simulink model "lab2_EmulationPID"  (R2020b)
settings: Solver=VariableStepAuto  StartTime=0.0  StopTime=10.0  RelTol=1e-3
undefined symbols (not defined in the file): denCdExact, denCdFE, denCdTustin, DiscIntNeverNeededParam, drv, enable_BlackBox, gbox, Kd, Ki, Kp, mld, mot, numCdExact, numCdFE, numCdTustin, rads2rpm, sens, stepAmplitude, tau_sf_hat_final, Tl, Ts
settings Model: Creator=Musta  LastModifiedBy=Musta

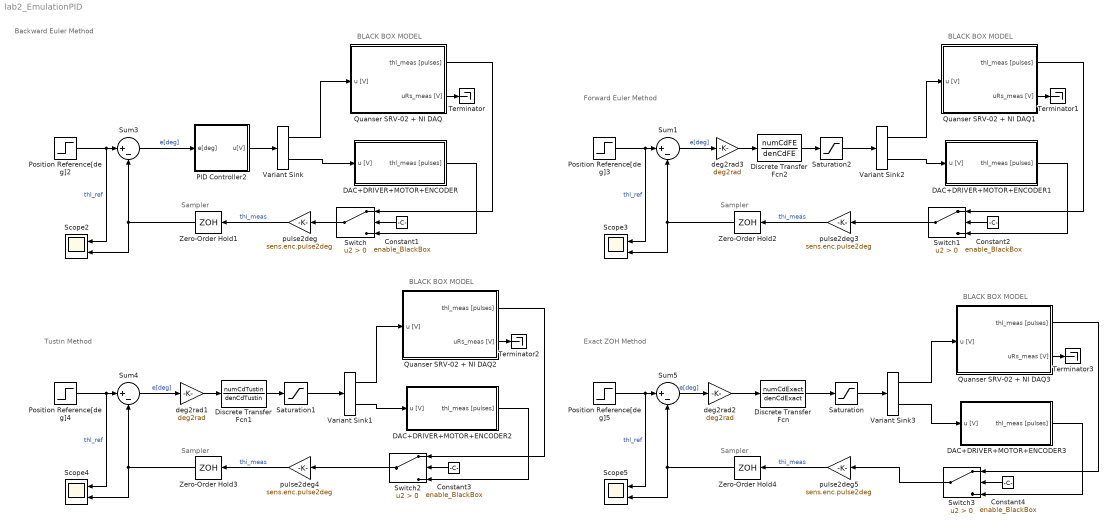
== system lab2_EmulationPID ==
  note: Tustin Method
  note: Sampler
  note: Sampler
  note: Forward Euler Method
  note: Backward Euler Method
  note: Sampler
  note: Sampler
  note: Exact ZOH Method
  note: BLACK BOX MODEL
  note: BLACK BOX MODEL
  note: BLACK BOX MODEL
  note: BLACK BOX MODEL
  Constant{1..4} (4 alike) : Constant  Value=enable_BlackBox
  DAC+DRIVER+MOTOR+ENCODER : Subsystem
  DAC+DRIVER+MOTOR+ENCODER1 : Subsystem
  DAC+DRIVER+MOTOR+ENCODER2 : Subsystem
  DAC+DRIVER+MOTOR+ENCODER3 : Subsystem
  Discrete Transfer Fcn : DiscreteTransferFcn  Numerator=numCdExact  Denominator=denCdExact  SampleTime=Ts
  Discrete Transfer Fcn1 : DiscreteTransferFcn  Numerator=numCdTustin  Denominator=denCdTustin  SampleTime=Ts
  Discrete Transfer Fcn2 : DiscreteTransferFcn  Numerator=numCdFE  Denominator=denCdFE  SampleTime=Ts
  PID Controller2 : Subsystem
  Position Reference[deg]{2..5} (4 alike) : Step  Time=0  After=stepAmplitude  SampleTime=0
  Quanser SRV-02 + NI DAQ : Subsystem  mask(Quanser SRV-02 (with inertial load) + NI DAQ){Ts=Ts, fricType=Karnopp}
      mask prompts: Ts "NI DAQ Sample Time:"; fricType "Friction model"
      mask help: Quanser SRV-02 (with inertial load) + NI DAQ model.
      mask init:
      | %%  Sensors data
      | 
      | %   shunt resistor
      | sens.curr.Rs = 0.5;                         %   resistance [Ohm]   
      | sens.curr.uRs_std = 0.01;                   %   voltage noise standard dev [V]                           
      | sens.curr.uRs_var = sens.curr.uRs_std^2;	%   voltage noise variance [V^2]
      | 
      | %   Hewlett-Packard HEDS-5540#A06 optical encoder
      | sens.enc.ppr = 500*4;                       %   pulses per rotation
      | sens.enc.pulse2deg = 360/sens.enc.ppr;      %   [pulses] -> [deg]
      | sens.enc.pulse2rad = 2*pi/sens.enc.ppr;     %   [pulses] -> [rad]
      | sens.enc.deg2pulse = sens.enc.ppr/360;      %   [deg] -> [pulses]
      | sens.enc.rad2pulse = sens.enc.ppr/2/pi;     %   [rad] -> [pulses]
      | 
      | 
      | %%  Data acquisition board (daq) data
      | 
      | %   NI PCI-6221 DAC data
      | daq.dac.bits = 16;                                  %   resolution (bits)
      | daq.dac.fs   = 10;                                  %   full scale 
      | daq.dac.q    = 2*daq.dac.fs/(2^daq.dac.bits-1);     %	quantization
      | 
      | %   NI PCI-6221 ADC data
      | daq.adc.bits = 16;                                  %   resolution (bits)
      | daq.adc.fs   = 10;                                  %   full scale (as set in SLDRT Analog Input block)
      | daq.adc.q    = 2*daq.adc.fs/(2^daq.adc.bits-1);     %   quantization
      mask Help:
      | Riccardo Antonello (antonello@dei.unipd.it)
      | 
      | April 24, 2020
      | 
      | Dept. of Information Engineering, University of Padova
      mask TypeOptions fricType: Coulomb + viscous | Karnopp
  Quanser SRV-02 + NI DAQ1 : Subsystem  mask(Quanser SRV-02 (with inertial load) + NI DAQ){Ts=Ts, fricType=Karnopp}
      mask prompts: Ts "NI DAQ Sample Time:"; fricType "Friction model"
      mask help: Quanser SRV-02 (with inertial load) + NI DAQ model.
      mask init: same as lab2_EmulationPID/Quanser SRV-02 + NI DAQ
      mask Help:
      | Riccardo Antonello (antonello@dei.unipd.it)
      | 
      | April 24, 2020
      | 
      | Dept. of Information Engineering, University of Padova
      mask TypeOptions fricType: Coulomb + viscous | Karnopp
  Quanser SRV-02 + NI DAQ2 : Subsystem  mask(Quanser SRV-02 (with inertial load) + NI DAQ){Ts=Ts, fricType=Karnopp}
      mask prompts: Ts "NI DAQ Sample Time:"; fricType "Friction model"
      mask help: Quanser SRV-02 (with inertial load) + NI DAQ model.
      mask init: same as lab2_EmulationPID/Quanser SRV-02 + NI DAQ
      mask Help:
      | Riccardo Antonello (antonello@dei.unipd.it)
      | 
      | April 24, 2020
      | 
      | Dept. of Information Engineering, University of Padova
      mask TypeOptions fricType: Coulomb + viscous | Karnopp
  Quanser SRV-02 + NI DAQ3 : Subsystem  mask(Quanser SRV-02 (with inertial load) + NI DAQ){Ts=Ts, fricType=Karnopp}
      mask prompts: Ts "NI DAQ Sample Time:"; fricType "Friction model"
      mask help: Quanser SRV-02 (with inertial load) + NI DAQ model.
      mask init: same as lab2_EmulationPID/Quanser SRV-02 + NI DAQ
      mask Help:
      | Riccardo Antonello (antonello@dei.unipd.it)
      | 
      | April 24, 2020
      | 
      | Dept. of Information Engineering, University of Padova
      mask TypeOptions fricType: Coulomb + viscous | Karnopp
  Saturation : Saturate  UpperLimit=10  LowerLimit=-10
  Saturation1 : Saturate  UpperLimit=10  LowerLimit=-10
  Saturation2 : Saturate  UpperLimit=10  LowerLimit=-10
  Scope{2..5} (4 alike) : Scope  NumInputPorts=2
  Sum{1,3..5} (4 alike) : Sum  Inputs=|+-
  Switch{,1..3} (4 alike) : Switch  Criteria=u2 > Threshold
  Terminator{,1..3} (4 alike) : Terminator
  Variant Sink{,1..3} (4 alike) : VariantSink
  Zero-Order Hold{1..4} (4 alike) : ZeroOrderHold  SampleTime=Ts
  deg2rad1 : Gain  Gain=deg2rad
  deg2rad2 : Gain  Gain=deg2rad
  deg2rad3 : Gain  Gain=deg2rad
  pulse2deg{,3..5} (4 alike) : Gain  Gain=sens.enc.pulse2deg
  wires:
  Position Reference[deg]3/1 -> Scope3/1, Sum1/1  "thl_ref"
  Position Reference[deg]5/1 -> Scope5/1, Sum5/1  "thl_ref"
  Sum5/1 -> deg2rad2/1  "e[deg]"
  Position Reference[deg]2/1 -> Scope2/1, Sum3/1  "thl_ref"
  pulse2deg3/1 -> Zero-Order Hold2/1  "thi_meas"
  Sum4/1 -> deg2rad1/1  "e[deg]"
  Zero-Order Hold3/1 -> Scope4/2, Sum4/2
  pulse2deg5/1 -> Zero-Order Hold4/1  "thi_meas"
  Zero-Order Hold2/1 -> Scope3/2, Sum1/2
  Saturation1/1 -> Variant Sink1/1
  Sum3/1 -> PID Controller2/1(e[deg])  "e[deg]"
  Zero-Order Hold1/1 -> Scope2/2, Sum3/2
  pulse2deg4/1 -> Zero-Order Hold3/1  "thi_meas"
  Zero-Order Hold4/1 -> Scope5/2, Sum5/2
  Discrete Transfer Fcn/1 -> Saturation/1
  Saturation/1 -> Variant Sink3/1
  deg2rad2/1 -> Discrete Transfer Fcn/1
  Position Reference[deg]4/1 -> Scope4/1, Sum4/1  "thl_ref"
  PID Controller2/1(u[V]) -> Variant Sink/1
  DAC+DRIVER+MOTOR+ENCODER/1(thl_meas [pulses]) -> Switch/3
  Variant Sink/2 -> DAC+DRIVER+MOTOR+ENCODER/1(u [V])
  Switch/1 -> pulse2deg/1
  Quanser SRV-02 + NI DAQ/1(thl_meas [pulses]) -> Switch/1
  pulse2deg/1 -> Zero-Order Hold1/1  "thi_meas"
  Quanser SRV-02 + NI DAQ/2(uRs_meas [V]) -> Terminator/1
  Variant Sink/1 -> Quanser SRV-02 + NI DAQ/1(u [V])
  Discrete Transfer Fcn1/1 -> Saturation1/1
  deg2rad1/1 -> Discrete Transfer Fcn1/1
  Saturation2/1 -> Variant Sink2/1
  deg2rad3/1 -> Discrete Transfer Fcn2/1
  Discrete Transfer Fcn2/1 -> Saturation2/1
  Sum1/1 -> deg2rad3/1  "e[deg]"
  Constant1/1 -> Switch/2
  Constant2/1 -> Switch1/2
  Quanser SRV-02 + NI DAQ1/1(thl_meas [pulses]) -> Switch1/1
  DAC+DRIVER+MOTOR+ENCODER1/1(thl_meas [pulses]) -> Switch1/3
  Variant Sink2/1 -> Quanser SRV-02 + NI DAQ1/1(u [V])
  Variant Sink2/2 -> DAC+DRIVER+MOTOR+ENCODER1/1(u [V])
  Quanser SRV-02 + NI DAQ1/2(uRs_meas [V]) -> Terminator1/1
  Switch1/1 -> pulse2deg3/1
  Constant3/1 -> Switch2/2
  Quanser SRV-02 + NI DAQ2/1(thl_meas [pulses]) -> Switch2/1
  DAC+DRIVER+MOTOR+ENCODER2/1(thl_meas [pulses]) -> Switch2/3
  Variant Sink1/1 -> Quanser SRV-02 + NI DAQ2/1(u [V])
  Variant Sink1/2 -> DAC+DRIVER+MOTOR+ENCODER2/1(u [V])
  Quanser SRV-02 + NI DAQ2/2(uRs_meas [V]) -> Terminator2/1
  Switch2/1 -> pulse2deg4/1
  Constant4/1 -> Switch3/2
  Quanser SRV-02 + NI DAQ3/1(thl_meas [pulses]) -> Switch3/1
  DAC+DRIVER+MOTOR+ENCODER3/1(thl_meas [pulses]) -> Switch3/3
  Variant Sink3/1 -> Quanser SRV-02 + NI DAQ3/1(u [V])
  Variant Sink3/2 -> DAC+DRIVER+MOTOR+ENCODER3/1(u [V])
  Quanser SRV-02 + NI DAQ3/2(uRs_meas [V]) -> Terminator3/1
  Switch3/1 -> pulse2deg5/1

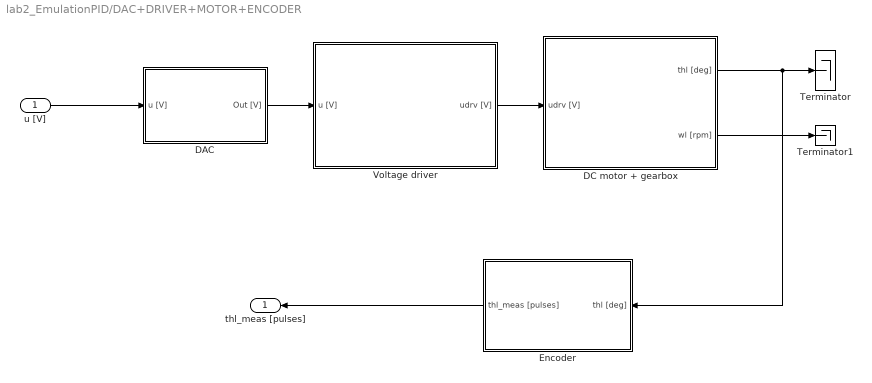
== system lab2_EmulationPID/DAC+DRIVER+MOTOR+ENCODER ==
  u [V] : Inport
  DAC : Subsystem
  DC motor + gearbox : Subsystem
  Encoder : Subsystem
  Terminator : Terminator
  Terminator1 : Terminator
  Voltage driver : Subsystem
  thl_meas [pulses] : Outport
  wires:
  DAC/1(Out [V]) -> Voltage driver/1(u [V])
  DC motor + gearbox/1("thl [deg] ") -> Terminator/1, Encoder/1("thl [deg] ")
  Voltage driver/1(udrv [V]) -> DC motor + gearbox/1(udrv [V])
  DC motor + gearbox/2(wl [rpm]) -> Terminator1/1
  Encoder/1(thl_meas [pulses]) -> thl_meas [pulses]/1
  u [V]/1 -> DAC/1(u [V])

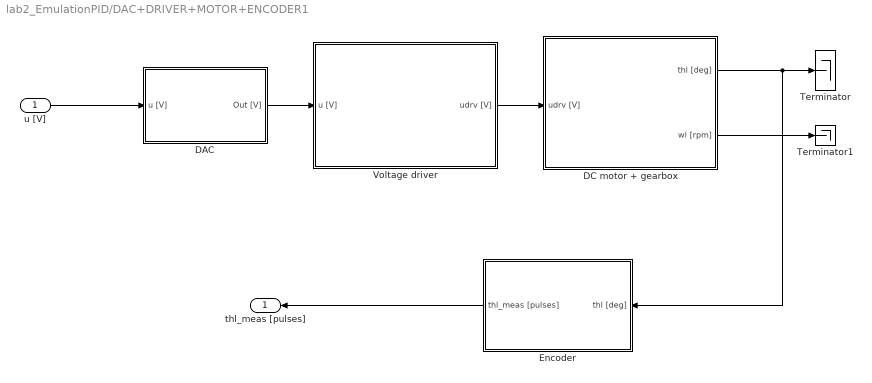
== system lab2_EmulationPID/DAC+DRIVER+MOTOR+ENCODER1 ==
  u [V] : Inport
  DAC : Subsystem
  DC motor + gearbox : Subsystem
  Encoder : Subsystem
  Terminator : Terminator
  Terminator1 : Terminator
  Voltage driver : Subsystem
  thl_meas [pulses] : Outport
  wires:
  DAC/1(Out [V]) -> Voltage driver/1(u [V])
  DC motor + gearbox/1("thl [deg] ") -> Terminator/1, Encoder/1("thl [deg] ")
  Voltage driver/1(udrv [V]) -> DC motor + gearbox/1(udrv [V])
  DC motor + gearbox/2(wl [rpm]) -> Terminator1/1
  Encoder/1(thl_meas [pulses]) -> thl_meas [pulses]/1
  u [V]/1 -> DAC/1(u [V])

== system lab2_EmulationPID/DAC+DRIVER+MOTOR+ENCODER2 ==
  u [V] : Inport
  DAC : Subsystem
  DC motor + gearbox : Subsystem
  Encoder : Subsystem
  Terminator : Terminator
  Terminator1 : Terminator
  Voltage driver : Subsystem
  thl_meas [pulses] : Outport
  wires:
  DAC/1(Out [V]) -> Voltage driver/1(u [V])
  DC motor + gearbox/1("thl [deg] ") -> Terminator/1, Encoder/1("thl [deg] ")
  Voltage driver/1(udrv [V]) -> DC motor + gearbox/1(udrv [V])
  DC motor + gearbox/2(wl [rpm]) -> Terminator1/1
  Encoder/1(thl_meas [pulses]) -> thl_meas [pulses]/1
  u [V]/1 -> DAC/1(u [V])

== system lab2_EmulationPID/DAC+DRIVER+MOTOR+ENCODER3 ==
  u [V] : Inport
  DAC : Subsystem
  DC motor + gearbox : Subsystem
  Encoder : Subsystem
  Terminator : Terminator
  Terminator1 : Terminator
  Voltage driver : Subsystem
  thl_meas [pulses] : Outport
  wires:
  DAC/1(Out [V]) -> Voltage driver/1(u [V])
  DC motor + gearbox/1("thl [deg] ") -> Terminator/1, Encoder/1("thl [deg] ")
  Voltage driver/1(udrv [V]) -> DC motor + gearbox/1(udrv [V])
  DC motor + gearbox/2(wl [rpm]) -> Terminator1/1
  Encoder/1(thl_meas [pulses]) -> thl_meas [pulses]/1
  u [V]/1 -> DAC/1(u [V])

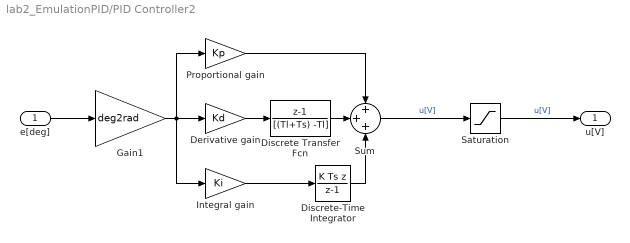
== system lab2_EmulationPID/PID Controller2 ==
  e[deg] : Inport
  Derivative gain : Gain  Gain=Kd
  Discrete Transfer Fcn : DiscreteTransferFcn  Numerator=[1 -1]  Denominator=[(Tl+Ts) -Tl]  SampleTime=Ts
  Discrete-Time Integrator : DiscreteIntegrator  IntegratorMethod=Integration: Backward Euler  SampleTime=Ts  ICPrevOutput=DiscIntNeverNeededParam  ICPrevScaledInput=DiscIntNeverNeededParam
  Gain1 : Gain  Gain=deg2rad
  Integral gain : Gain  Gain=Ki
  Proportional gain : Gain  Gain=Kp
  Saturation : Saturate  UpperLimit=10  LowerLimit=-10
  Sum : Sum  Inputs=+++
  u[V] : Outport
  wires:
  e[deg]/1 -> Gain1/1
  Discrete Transfer Fcn/1 -> Sum/2
  Gain1/1 -> Proportional gain/1, Integral gain/1, Derivative gain/1
  Proportional gain/1 -> Sum/1
  Discrete-Time Integrator/1 -> Sum/3
  Derivative gain/1 -> Discrete Transfer Fcn/1
  Saturation/1 -> u[V]/1  "u[V]"
  Sum/1 -> Saturation/1  "u[V]"
  Integral gain/1 -> Discrete-Time Integrator/1

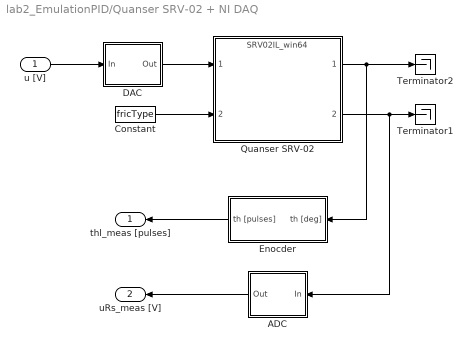
== system lab2_EmulationPID/Quanser SRV-02 + NI DAQ ==
  u [V] : Inport
  ADC : Subsystem
  Constant : Constant  Value=fricType
  DAC : Subsystem
  Enocder : Subsystem
  Quanser SRV-02 : ModelReference  ModelNameDialog=SRV02IL_win64.slxp  ModelReferenceVersion=1.44  CopyOfModelProtected=on
  Terminator1 : Terminator
  Terminator2 : Terminator
  thl_meas [pulses] : Outport
  uRs_meas [V] : Outport  Port=2
  wires:
  Enocder/1(th [pulses]) -> thl_meas [pulses]/1
  ADC/1(Out) -> uRs_meas [V]/1
  DAC/1(Out) -> Quanser SRV-02/1
  Quanser SRV-02/2 -> ADC/1(In), Terminator1/1
  u [V]/1 -> DAC/1(In)
  Quanser SRV-02/1 -> Enocder/1(th [deg]), Terminator2/1
  Constant/1 -> Quanser SRV-02/2

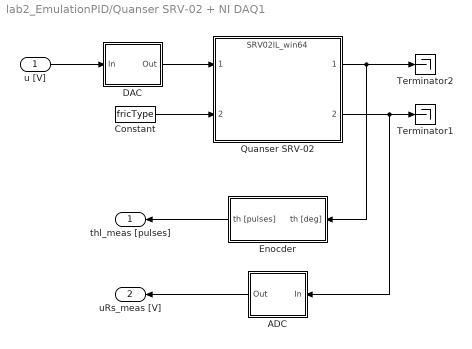
== system lab2_EmulationPID/Quanser SRV-02 + NI DAQ1 ==
  u [V] : Inport
  ADC : Subsystem
  Constant : Constant  Value=fricType
  DAC : Subsystem
  Enocder : Subsystem
  Quanser SRV-02 : ModelReference  ModelNameDialog=SRV02IL_win64.slxp  ModelReferenceVersion=1.44  CopyOfModelProtected=on
  Terminator1 : Terminator
  Terminator2 : Terminator
  thl_meas [pulses] : Outport
  uRs_meas [V] : Outport  Port=2
  wires:
  Enocder/1(th [pulses]) -> thl_meas [pulses]/1
  ADC/1(Out) -> uRs_meas [V]/1
  DAC/1(Out) -> Quanser SRV-02/1
  Quanser SRV-02/2 -> ADC/1(In), Terminator1/1
  u [V]/1 -> DAC/1(In)
  Quanser SRV-02/1 -> Enocder/1(th [deg]), Terminator2/1
  Constant/1 -> Quanser SRV-02/2

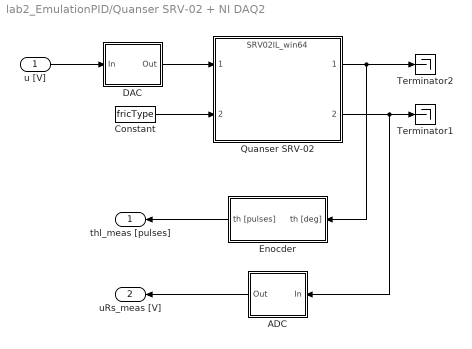
== system lab2_EmulationPID/Quanser SRV-02 + NI DAQ2 ==
  u [V] : Inport
  ADC : Subsystem
  Constant : Constant  Value=fricType
  DAC : Subsystem
  Enocder : Subsystem
  Quanser SRV-02 : ModelReference  ModelNameDialog=SRV02IL_win64.slxp  ModelReferenceVersion=1.44  CopyOfModelProtected=on
  Terminator1 : Terminator
  Terminator2 : Terminator
  thl_meas [pulses] : Outport
  uRs_meas [V] : Outport  Port=2
  wires:
  Enocder/1(th [pulses]) -> thl_meas [pulses]/1
  ADC/1(Out) -> uRs_meas [V]/1
  DAC/1(Out) -> Quanser SRV-02/1
  Quanser SRV-02/2 -> ADC/1(In), Terminator1/1
  u [V]/1 -> DAC/1(In)
  Quanser SRV-02/1 -> Enocder/1(th [deg]), Terminator2/1
  Constant/1 -> Quanser SRV-02/2

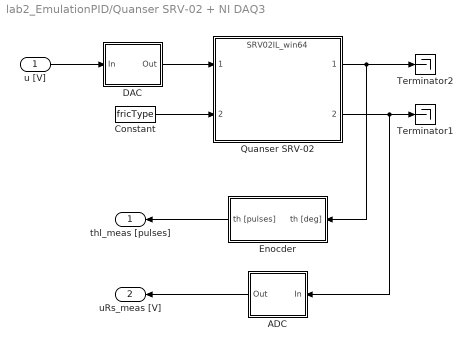
== system lab2_EmulationPID/Quanser SRV-02 + NI DAQ3 ==
  u [V] : Inport
  ADC : Subsystem
  Constant : Constant  Value=fricType
  DAC : Subsystem
  Enocder : Subsystem
  Quanser SRV-02 : ModelReference  ModelNameDialog=SRV02IL_win64.slxp  ModelReferenceVersion=1.44  CopyOfModelProtected=on
  Terminator1 : Terminator
  Terminator2 : Terminator
  thl_meas [pulses] : Outport
  uRs_meas [V] : Outport  Port=2
  wires:
  Enocder/1(th [pulses]) -> thl_meas [pulses]/1
  ADC/1(Out) -> uRs_meas [V]/1
  DAC/1(Out) -> Quanser SRV-02/1
  Quanser SRV-02/2 -> ADC/1(In), Terminator1/1
  u [V]/1 -> DAC/1(In)
  Quanser SRV-02/1 -> Enocder/1(th [deg]), Terminator2/1
  Constant/1 -> Quanser SRV-02/2

== system lab2_EmulationPID/DAC+DRIVER+MOTOR+ENCODER/DAC ==
  u [V] : Inport
  Quantizer : Quantizer  QuantizationInterval=20/(2^16-1)
  Saturation : Saturate  UpperLimit=10  LowerLimit=-10
  Zero-Order Hold : ZeroOrderHold  SampleTime=Ts
  Out [V] : Outport
  wires:
  u [V]/1 -> Zero-Order Hold/1
  Zero-Order Hold/1 -> Quantizer/1
  Quantizer/1 -> Saturation/1
  Saturation/1 -> Out [V]/1

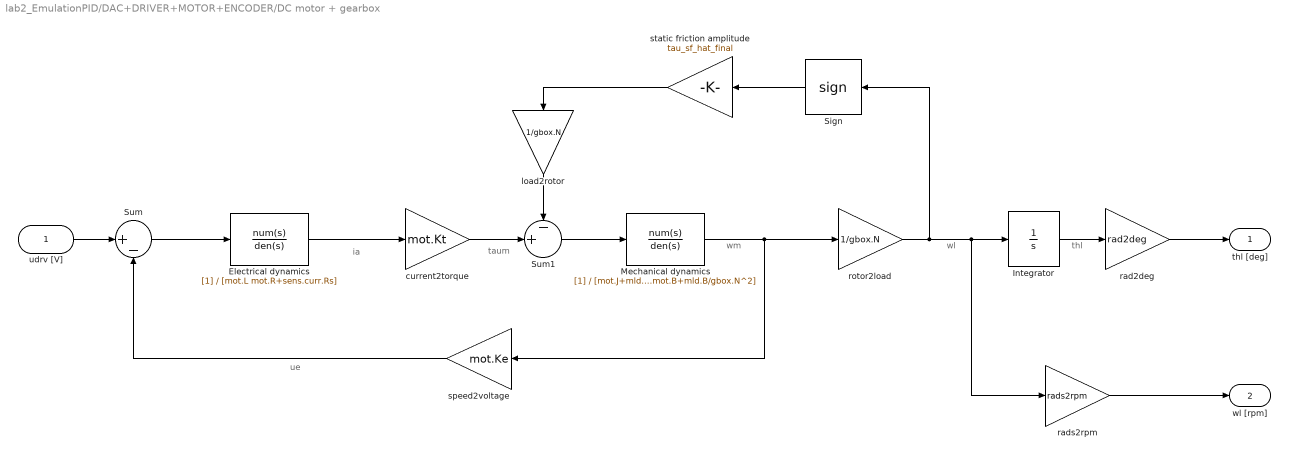
== system lab2_EmulationPID/DAC+DRIVER+MOTOR+ENCODER/DC motor + gearbox ==
  note: thl
  note: wl
  note: wm
  note: ue
  note: taum
  note: ia
  udrv [V] : Inport
  Electrical dynamics : TransferFcn  Denominator=[mot.L mot.R+sens.curr.Rs]
  Integrator : Integrator
  Mechanical dynamics : TransferFcn  Denominator=[mot.J+mld.J/gbox.N^2 mot.B+mld.B/gbox.N^2]
  Sign : Signum  ZeroCross=off
  Sum : Sum  Inputs=|+-
  Sum1 : Sum  Inputs=-+|
  current2torque : Gain  Gain=mot.Kt
  load2rotor : Gain  Gain=1/gbox.N
  rad2deg : Gain  Gain=rad2deg
  rads2rpm : Gain  Gain=rads2rpm
  rotor2load : Gain  Gain=1/gbox.N
  speed2voltage : Gain  Gain=mot.Ke
  static friction amplitude : Gain  Gain=tau_sf_hat_final
  "thl [deg] " : Outport
  wl [rpm] : Outport  Port=2
  wires:
  static friction amplitude/1 -> load2rotor/1
  udrv [V]/1 -> Sum/1
  Electrical dynamics/1 -> current2torque/1
  current2torque/1 -> Sum1/2
  load2rotor/1 -> Sum1/1
  Sign/1 -> static friction amplitude/1
  speed2voltage/1 -> Sum/2
  rad2deg/1 -> "thl [deg] "/1
  Sum1/1 -> Mechanical dynamics/1
  Mechanical dynamics/1 -> speed2voltage/1, rotor2load/1
  rads2rpm/1 -> wl [rpm]/1
  Sum/1 -> Electrical dynamics/1
  rotor2load/1 -> Sign/1, rads2rpm/1, Integrator/1
  Integrator/1 -> rad2deg/1

== system lab2_EmulationPID/DAC+DRIVER+MOTOR+ENCODER/Encoder ==
  "thl [deg] " : Inport
  Gain : Gain  Gain=2000/360
  Quantizer : Quantizer  QuantizationInterval=360/(500*4)
  Zero-Order Hold : ZeroOrderHold  SampleTime=Ts
  thl_meas [pulses] : Outport
  wires:
  "thl [deg] "/1 -> Zero-Order Hold/1
  Zero-Order Hold/1 -> Quantizer/1
  Quantizer/1 -> Gain/1
  Gain/1 -> thl_meas [pulses]/1

== system lab2_EmulationPID/DAC+DRIVER+MOTOR+ENCODER/Voltage driver ==
  u [V] : Inport
  Saturation : Saturate  UpperLimit=10  LowerLimit=-10
  Transfer Fcn : TransferFcn  Numerator=[drv.dcgain]  Denominator=[drv.Tc 1]
  udrv [V] : Outport
  wires:
  u [V]/1 -> Transfer Fcn/1
  Transfer Fcn/1 -> Saturation/1
  Saturation/1 -> udrv [V]/1

== system lab2_EmulationPID/DAC+DRIVER+MOTOR+ENCODER1/DAC ==
  u [V] : Inport
  Quantizer : Quantizer  QuantizationInterval=20/(2^16-1)
  Saturation : Saturate  UpperLimit=10  LowerLimit=-10
  Zero-Order Hold : ZeroOrderHold  SampleTime=Ts
  Out [V] : Outport
  wires:
  u [V]/1 -> Zero-Order Hold/1
  Zero-Order Hold/1 -> Quantizer/1
  Quantizer/1 -> Saturation/1
  Saturation/1 -> Out [V]/1

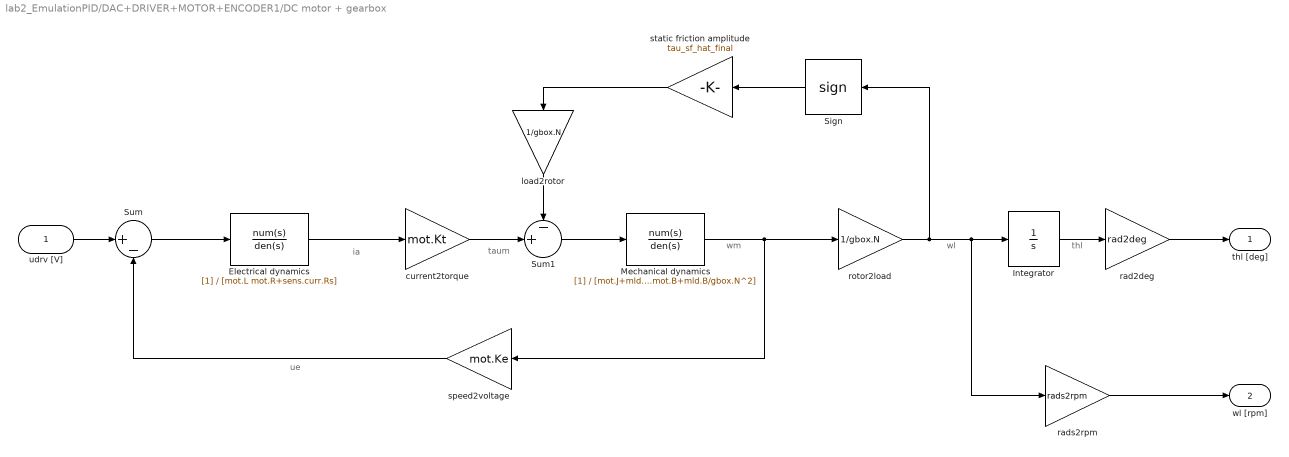
== system lab2_EmulationPID/DAC+DRIVER+MOTOR+ENCODER1/DC motor + gearbox ==
  note: thl
  note: wl
  note: wm
  note: ue
  note: taum
  note: ia
  udrv [V] : Inport
  Electrical dynamics : TransferFcn  Denominator=[mot.L mot.R+sens.curr.Rs]
  Integrator : Integrator
  Mechanical dynamics : TransferFcn  Denominator=[mot.J+mld.J/gbox.N^2 mot.B+mld.B/gbox.N^2]
  Sign : Signum  ZeroCross=off
  Sum : Sum  Inputs=|+-
  Sum1 : Sum  Inputs=-+|
  current2torque : Gain  Gain=mot.Kt
  load2rotor : Gain  Gain=1/gbox.N
  rad2deg : Gain  Gain=rad2deg
  rads2rpm : Gain  Gain=rads2rpm
  rotor2load : Gain  Gain=1/gbox.N
  speed2voltage : Gain  Gain=mot.Ke
  static friction amplitude : Gain  Gain=tau_sf_hat_final
  "thl [deg] " : Outport
  wl [rpm] : Outport  Port=2
  wires:
  static friction amplitude/1 -> load2rotor/1
  udrv [V]/1 -> Sum/1
  Electrical dynamics/1 -> current2torque/1
  current2torque/1 -> Sum1/2
  load2rotor/1 -> Sum1/1
  Sign/1 -> static friction amplitude/1
  speed2voltage/1 -> Sum/2
  rad2deg/1 -> "thl [deg] "/1
  Sum1/1 -> Mechanical dynamics/1
  Mechanical dynamics/1 -> speed2voltage/1, rotor2load/1
  rads2rpm/1 -> wl [rpm]/1
  Sum/1 -> Electrical dynamics/1
  rotor2load/1 -> Sign/1, rads2rpm/1, Integrator/1
  Integrator/1 -> rad2deg/1

== system lab2_EmulationPID/DAC+DRIVER+MOTOR+ENCODER1/Encoder ==
  "thl [deg] " : Inport
  Gain : Gain  Gain=2000/360
  Quantizer : Quantizer  QuantizationInterval=360/(500*4)
  Zero-Order Hold : ZeroOrderHold  SampleTime=Ts
  thl_meas [pulses] : Outport
  wires:
  "thl [deg] "/1 -> Zero-Order Hold/1
  Zero-Order Hold/1 -> Quantizer/1
  Quantizer/1 -> Gain/1
  Gain/1 -> thl_meas [pulses]/1

== system lab2_EmulationPID/DAC+DRIVER+MOTOR+ENCODER1/Voltage driver ==
  u [V] : Inport
  Saturation : Saturate  UpperLimit=10  LowerLimit=-10
  Transfer Fcn : TransferFcn  Numerator=[drv.dcgain]  Denominator=[drv.Tc 1]
  udrv [V] : Outport
  wires:
  u [V]/1 -> Transfer Fcn/1
  Transfer Fcn/1 -> Saturation/1
  Saturation/1 -> udrv [V]/1

== system lab2_EmulationPID/DAC+DRIVER+MOTOR+ENCODER2/DAC ==
  u [V] : Inport
  Quantizer : Quantizer  QuantizationInterval=20/(2^16-1)
  Saturation : Saturate  UpperLimit=10  LowerLimit=-10
  Zero-Order Hold : ZeroOrderHold  SampleTime=Ts
  Out [V] : Outport
  wires:
  u [V]/1 -> Zero-Order Hold/1
  Zero-Order Hold/1 -> Quantizer/1
  Quantizer/1 -> Saturation/1
  Saturation/1 -> Out [V]/1

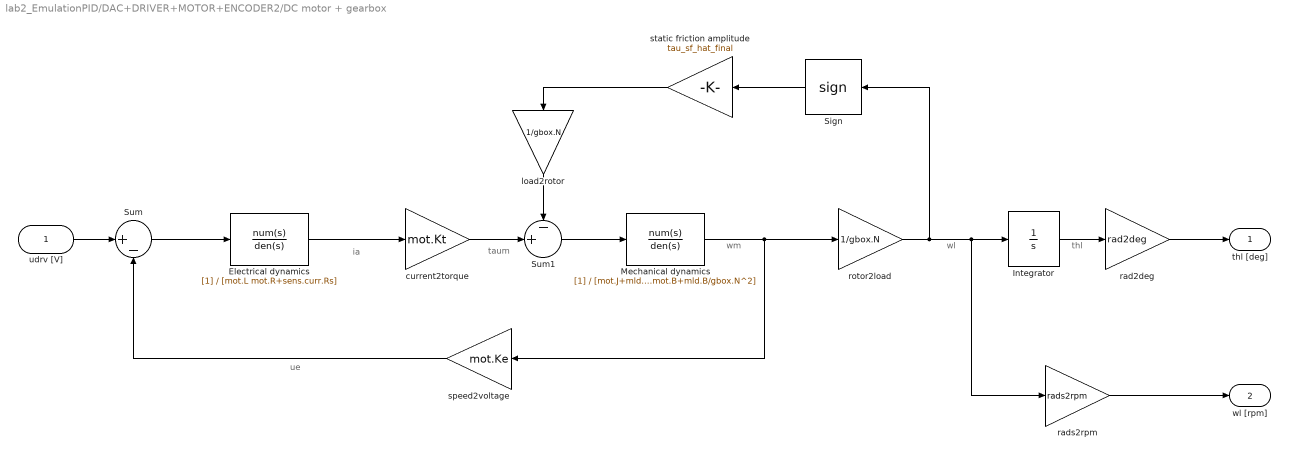
== system lab2_EmulationPID/DAC+DRIVER+MOTOR+ENCODER2/DC motor + gearbox ==
  note: thl
  note: wl
  note: wm
  note: ue
  note: taum
  note: ia
  udrv [V] : Inport
  Electrical dynamics : TransferFcn  Denominator=[mot.L mot.R+sens.curr.Rs]
  Integrator : Integrator
  Mechanical dynamics : TransferFcn  Denominator=[mot.J+mld.J/gbox.N^2 mot.B+mld.B/gbox.N^2]
  Sign : Signum  ZeroCross=off
  Sum : Sum  Inputs=|+-
  Sum1 : Sum  Inputs=-+|
  current2torque : Gain  Gain=mot.Kt
  load2rotor : Gain  Gain=1/gbox.N
  rad2deg : Gain  Gain=rad2deg
  rads2rpm : Gain  Gain=rads2rpm
  rotor2load : Gain  Gain=1/gbox.N
  speed2voltage : Gain  Gain=mot.Ke
  static friction amplitude : Gain  Gain=tau_sf_hat_final
  "thl [deg] " : Outport
  wl [rpm] : Outport  Port=2
  wires:
  static friction amplitude/1 -> load2rotor/1
  udrv [V]/1 -> Sum/1
  Electrical dynamics/1 -> current2torque/1
  current2torque/1 -> Sum1/2
  load2rotor/1 -> Sum1/1
  Sign/1 -> static friction amplitude/1
  speed2voltage/1 -> Sum/2
  rad2deg/1 -> "thl [deg] "/1
  Sum1/1 -> Mechanical dynamics/1
  Mechanical dynamics/1 -> speed2voltage/1, rotor2load/1
  rads2rpm/1 -> wl [rpm]/1
  Sum/1 -> Electrical dynamics/1
  rotor2load/1 -> Sign/1, rads2rpm/1, Integrator/1
  Integrator/1 -> rad2deg/1

== system lab2_EmulationPID/DAC+DRIVER+MOTOR+ENCODER2/Encoder ==
  "thl [deg] " : Inport
  Gain : Gain  Gain=2000/360
  Quantizer : Quantizer  QuantizationInterval=360/(500*4)
  Zero-Order Hold : ZeroOrderHold  SampleTime=Ts
  thl_meas [pulses] : Outport
  wires:
  "thl [deg] "/1 -> Zero-Order Hold/1
  Zero-Order Hold/1 -> Quantizer/1
  Quantizer/1 -> Gain/1
  Gain/1 -> thl_meas [pulses]/1

== system lab2_EmulationPID/DAC+DRIVER+MOTOR+ENCODER2/Voltage driver ==
  u [V] : Inport
  Saturation : Saturate  UpperLimit=10  LowerLimit=-10
  Transfer Fcn : TransferFcn  Numerator=[drv.dcgain]  Denominator=[drv.Tc 1]
  udrv [V] : Outport
  wires:
  u [V]/1 -> Transfer Fcn/1
  Transfer Fcn/1 -> Saturation/1
  Saturation/1 -> udrv [V]/1

== system lab2_EmulationPID/DAC+DRIVER+MOTOR+ENCODER3/DAC ==
  u [V] : Inport
  Quantizer : Quantizer  QuantizationInterval=20/(2^16-1)
  Saturation : Saturate  UpperLimit=10  LowerLimit=-10
  Zero-Order Hold : ZeroOrderHold  SampleTime=Ts
  Out [V] : Outport
  wires:
  u [V]/1 -> Zero-Order Hold/1
  Zero-Order Hold/1 -> Quantizer/1
  Quantizer/1 -> Saturation/1
  Saturation/1 -> Out [V]/1

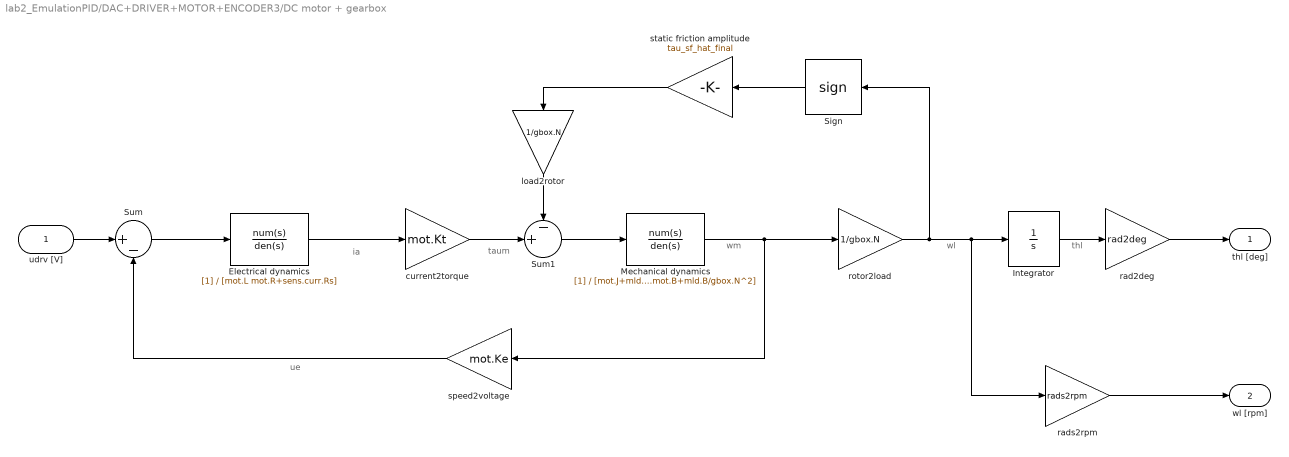
== system lab2_EmulationPID/DAC+DRIVER+MOTOR+ENCODER3/DC motor + gearbox ==
  note: thl
  note: wl
  note: wm
  note: ue
  note: taum
  note: ia
  udrv [V] : Inport
  Electrical dynamics : TransferFcn  Denominator=[mot.L mot.R+sens.curr.Rs]
  Integrator : Integrator
  Mechanical dynamics : TransferFcn  Denominator=[mot.J+mld.J/gbox.N^2 mot.B+mld.B/gbox.N^2]
  Sign : Signum  ZeroCross=off
  Sum : Sum  Inputs=|+-
  Sum1 : Sum  Inputs=-+|
  current2torque : Gain  Gain=mot.Kt
  load2rotor : Gain  Gain=1/gbox.N
  rad2deg : Gain  Gain=rad2deg
  rads2rpm : Gain  Gain=rads2rpm
  rotor2load : Gain  Gain=1/gbox.N
  speed2voltage : Gain  Gain=mot.Ke
  static friction amplitude : Gain  Gain=tau_sf_hat_final
  "thl [deg] " : Outport
  wl [rpm] : Outport  Port=2
  wires:
  static friction amplitude/1 -> load2rotor/1
  udrv [V]/1 -> Sum/1
  Electrical dynamics/1 -> current2torque/1
  current2torque/1 -> Sum1/2
  load2rotor/1 -> Sum1/1
  Sign/1 -> static friction amplitude/1
  speed2voltage/1 -> Sum/2
  rad2deg/1 -> "thl [deg] "/1
  Sum1/1 -> Mechanical dynamics/1
  Mechanical dynamics/1 -> speed2voltage/1, rotor2load/1
  rads2rpm/1 -> wl [rpm]/1
  Sum/1 -> Electrical dynamics/1
  rotor2load/1 -> Sign/1, rads2rpm/1, Integrator/1
  Integrator/1 -> rad2deg/1

== system lab2_EmulationPID/DAC+DRIVER+MOTOR+ENCODER3/Encoder ==
  "thl [deg] " : Inport
  Gain : Gain  Gain=2000/360
  Quantizer : Quantizer  QuantizationInterval=360/(500*4)
  Zero-Order Hold : ZeroOrderHold  SampleTime=Ts
  thl_meas [pulses] : Outport
  wires:
  "thl [deg] "/1 -> Zero-Order Hold/1
  Zero-Order Hold/1 -> Quantizer/1
  Quantizer/1 -> Gain/1
  Gain/1 -> thl_meas [pulses]/1

== system lab2_EmulationPID/DAC+DRIVER+MOTOR+ENCODER3/Voltage driver ==
  u [V] : Inport
  Saturation : Saturate  UpperLimit=10  LowerLimit=-10
  Transfer Fcn : TransferFcn  Numerator=[drv.dcgain]  Denominator=[drv.Tc 1]
  udrv [V] : Outport
  wires:
  u [V]/1 -> Transfer Fcn/1
  Transfer Fcn/1 -> Saturation/1
  Saturation/1 -> udrv [V]/1

== system lab2_EmulationPID/Quanser SRV-02 + NI DAQ/ADC ==
  In : Inport
  Quantizer : Quantizer  QuantizationInterval=daq.adc.q
  Saturation : Saturate  UpperLimit=daq.adc.fs  LowerLimit=-daq.adc.fs
  Zero-Order Hold : ZeroOrderHold  SampleTime=Ts
  Out : Outport
  wires:
  Saturation/1 -> Out/1
  In/1 -> Zero-Order Hold/1
  Quantizer/1 -> Saturation/1
  Zero-Order Hold/1 -> Quantizer/1

== system lab2_EmulationPID/Quanser SRV-02 + NI DAQ/DAC ==
  In : Inport
  Quantizer : Quantizer  QuantizationInterval=daq.dac.q
  Saturation : Saturate  UpperLimit=daq.dac.fs  LowerLimit=-daq.dac.fs
  Zero-Order Hold : ZeroOrderHold  SampleTime=Ts
  Out : Outport
  wires:
  Quantizer/1 -> Saturation/1
  In/1 -> Zero-Order Hold/1
  Zero-Order Hold/1 -> Quantizer/1
  Saturation/1 -> Out/1

== system lab2_EmulationPID/Quanser SRV-02 + NI DAQ/Enocder ==
  th [deg] : Inport
  Quantizer : Quantizer  QuantizationInterval=sens.enc.pulse2deg
  Zero-Order Hold : ZeroOrderHold  SampleTime=Ts
  deg2pulse : Gain  Gain=sens.enc.deg2pulse
  th [pulses] : Outport
  wires:
  Quantizer/1 -> deg2pulse/1
  th [deg]/1 -> Zero-Order Hold/1
  Zero-Order Hold/1 -> Quantizer/1
  deg2pulse/1 -> th [pulses]/1

== system lab2_EmulationPID/Quanser SRV-02 + NI DAQ1/ADC ==
  In : Inport
  Quantizer : Quantizer  QuantizationInterval=daq.adc.q
  Saturation : Saturate  UpperLimit=daq.adc.fs  LowerLimit=-daq.adc.fs
  Zero-Order Hold : ZeroOrderHold  SampleTime=Ts
  Out : Outport
  wires:
  Saturation/1 -> Out/1
  In/1 -> Zero-Order Hold/1
  Quantizer/1 -> Saturation/1
  Zero-Order Hold/1 -> Quantizer/1

== system lab2_EmulationPID/Quanser SRV-02 + NI DAQ1/DAC ==
  In : Inport
  Quantizer : Quantizer  QuantizationInterval=daq.dac.q
  Saturation : Saturate  UpperLimit=daq.dac.fs  LowerLimit=-daq.dac.fs
  Zero-Order Hold : ZeroOrderHold  SampleTime=Ts
  Out : Outport
  wires:
  Quantizer/1 -> Saturation/1
  In/1 -> Zero-Order Hold/1
  Zero-Order Hold/1 -> Quantizer/1
  Saturation/1 -> Out/1

== system lab2_EmulationPID/Quanser SRV-02 + NI DAQ1/Enocder ==
  th [deg] : Inport
  Quantizer : Quantizer  QuantizationInterval=sens.enc.pulse2deg
  Zero-Order Hold : ZeroOrderHold  SampleTime=Ts
  deg2pulse : Gain  Gain=sens.enc.deg2pulse
  th [pulses] : Outport
  wires:
  Quantizer/1 -> deg2pulse/1
  th [deg]/1 -> Zero-Order Hold/1
  Zero-Order Hold/1 -> Quantizer/1
  deg2pulse/1 -> th [pulses]/1

== system lab2_EmulationPID/Quanser SRV-02 + NI DAQ2/ADC ==
  In : Inport
  Quantizer : Quantizer  QuantizationInterval=daq.adc.q
  Saturation : Saturate  UpperLimit=daq.adc.fs  LowerLimit=-daq.adc.fs
  Zero-Order Hold : ZeroOrderHold  SampleTime=Ts
  Out : Outport
  wires:
  Saturation/1 -> Out/1
  In/1 -> Zero-Order Hold/1
  Quantizer/1 -> Saturation/1
  Zero-Order Hold/1 -> Quantizer/1

== system lab2_EmulationPID/Quanser SRV-02 + NI DAQ2/DAC ==
  In : Inport
  Quantizer : Quantizer  QuantizationInterval=daq.dac.q
  Saturation : Saturate  UpperLimit=daq.dac.fs  LowerLimit=-daq.dac.fs
  Zero-Order Hold : ZeroOrderHold  SampleTime=Ts
  Out : Outport
  wires:
  Quantizer/1 -> Saturation/1
  In/1 -> Zero-Order Hold/1
  Zero-Order Hold/1 -> Quantizer/1
  Saturation/1 -> Out/1

== system lab2_EmulationPID/Quanser SRV-02 + NI DAQ2/Enocder ==
  th [deg] : Inport
  Quantizer : Quantizer  QuantizationInterval=sens.enc.pulse2deg
  Zero-Order Hold : ZeroOrderHold  SampleTime=Ts
  deg2pulse : Gain  Gain=sens.enc.deg2pulse
  th [pulses] : Outport
  wires:
  Quantizer/1 -> deg2pulse/1
  th [deg]/1 -> Zero-Order Hold/1
  Zero-Order Hold/1 -> Quantizer/1
  deg2pulse/1 -> th [pulses]/1

== system lab2_EmulationPID/Quanser SRV-02 + NI DAQ3/ADC ==
  In : Inport
  Quantizer : Quantizer  QuantizationInterval=daq.adc.q
  Saturation : Saturate  UpperLimit=daq.adc.fs  LowerLimit=-daq.adc.fs
  Zero-Order Hold : ZeroOrderHold  SampleTime=Ts
  Out : Outport
  wires:
  Saturation/1 -> Out/1
  In/1 -> Zero-Order Hold/1
  Quantizer/1 -> Saturation/1
  Zero-Order Hold/1 -> Quantizer/1

== system lab2_EmulationPID/Quanser SRV-02 + NI DAQ3/DAC ==
  In : Inport
  Quantizer : Quantizer  QuantizationInterval=daq.dac.q
  Saturation : Saturate  UpperLimit=daq.dac.fs  LowerLimit=-daq.dac.fs
  Zero-Order Hold : ZeroOrderHold  SampleTime=Ts
  Out : Outport
  wires:
  Quantizer/1 -> Saturation/1
  In/1 -> Zero-Order Hold/1
  Zero-Order Hold/1 -> Quantizer/1
  Saturation/1 -> Out/1

== system lab2_EmulationPID/Quanser SRV-02 + NI DAQ3/Enocder ==
  th [deg] : Inport
  Quantizer : Quantizer  QuantizationInterval=sens.enc.pulse2deg
  Zero-Order Hold : ZeroOrderHold  SampleTime=Ts
  deg2pulse : Gain  Gain=sens.enc.deg2pulse
  th [pulses] : Outport
  wires:
  Quantizer/1 -> deg2pulse/1
  th [deg]/1 -> Zero-Order Hold/1
  Zero-Order Hold/1 -> Quantizer/1
  deg2pulse/1 -> th [pulses]/1
